simulink model "ss_model"  (Simulink 7.5)
settings: Solver=ode23s  StartTime=0.0  StopTime=300  RelTol=1e-3
values from neighbouring files (symbols this model uses):
  A = [ ... (first row only)    [vodarna_diff.m]    (also in vodarna_diff_ser.m)
  B = [u; 0; 0; 0; 0; 0]    [vodarna_diff.m]
  C = eye(6)    [vodarna_diff.m]
  D = [0; 0; 0; 0; 0; 0]    [vodarna_diff.m]
  x0 = [0 0 0 10 0 0]    [vodarna_diff.m]
settings Model: Creator=michal  LastModifiedBy=michal

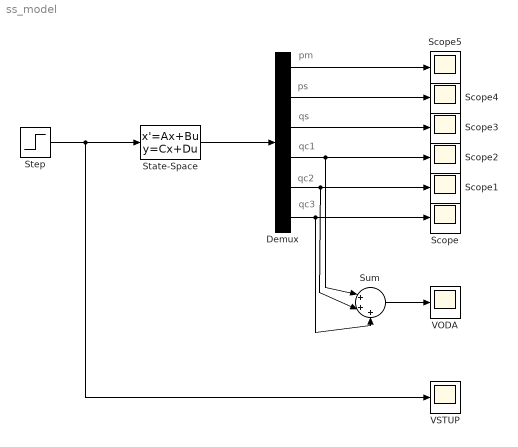
== system ss_model ==
  note: pm
  note: ps
  note: qs
  note: qc1
  note: qc2
  note: qc3
  Demux : Demux  Outputs=6
  Scope{,1..5} (6 alike) : Scope
      Scope1 settings: YMin=0  YMax=140000
      Scope2 settings: SaveName=ScopeData2
      Scope3 settings: SaveName=ScopeData3
      Scope4 settings: SaveName=ScopeData4
      Scope5 settings: SaveName=ScopeData5
  State-Space : StateSpace  A=A  B=B  C=C  D=D  X0=x0
  Step : Step  Time=230  Before=1  After=0  SampleTime=0
  Sum : Sum  Inputs=|+++  OutDataType=fixdt(1, 16)  OutScaling=2^0
  VODA : Scope
      settings: DataFormat=Array
  VSTUP : Scope
      settings: SaveName=ScopeData7
  wires:
  Step/1 -> State-Space/1, VSTUP/1
  State-Space/1 -> Demux/1
  Demux/1 -> Scope5/1
  Demux/2 -> Scope4/1
  Demux/3 -> Scope3/1
  Demux/4 -> Scope2/1, Sum/1
  Demux/5 -> Scope1/1, Sum/2
  Demux/6 -> Scope/1, Sum/3
  Sum/1 -> VODA/1
